simulink model "CrCtl_Governor"  (R2016b)
settings: configuration reference "CodeGenConfigSet" (kept outside this file)
values from neighbouring files (symbols this model uses):
  ACC_ZERO = fi(0,Acc_m_s2)    [init_CrCtl_Governor.m]
  CrCtl_facAcc2TrqCor_C = Calibration.Parameter    [init_CrCtl_Governor.m]
  CrCtl_facDecl2TrqCor_C = Calibration.Parameter    [init_CrCtl_Governor.m]
  CrCtl_facPT11_C = Calibration.Parameter    [init_CrCtl_Governor.m]
  CrCtl_facPT12_C = Calibration.Parameter    [init_CrCtl_Governor.m]
  CrCtl_facPT13_C = Calibration.Parameter    [init_CrCtl_Governor.m]
  CrCtl_facRmpSlpHiAcc_C = Calibration.Parameter    [init_CrCtl_Governor.m]
  CrCtl_facRmpSlpHiDecl_C = Calibration.Parameter    [init_CrCtl_Governor.m]
  CrCtl_facSlpConstRmpDwn_C = Calibration.Parameter    [init_CrCtl_Governor.m]
  CrCtl_facSlpConstRmpUp_C = Calibration.Parameter    [init_CrCtl_Governor.m]
  CrCtl_facSlpRmp1Sus_C = Calibration.Parameter    [init_CrCtl_Governor.m]
  CrCtl_facSlpRmp2Sus_C = Calibration.Parameter    [init_CrCtl_Governor.m]
  CrCtl_facTipDwnCor_CUR = Calibration.Parameter    [init_CrCtl_Governor.m]
  CrCtl_facTipDwnCor_CURX = Calibration.Parameter    [init_CrCtl_Governor.m]
  CrCtl_facTipUpCor_CUR = Calibration.Parameter    [init_CrCtl_Governor.m]
  CrCtl_facTipUpCor_CURX = Calibration.Parameter    [init_CrCtl_Governor.m]
  CrCtl_facTrqIncrSlpConstRmp_C = Calibration.Parameter    [init_CrCtl_Governor.m]
  CrCtl_facTrqIncrTimeConstRmp_C = Calibration.Parameter    [init_CrCtl_Governor.m]
  CrCtl_facTrqRedSlpConstRmp_C = Calibration.Parameter    [init_CrCtl_Governor.m]
  CrCtl_facTrqRedTimeConstRmp_C = Calibration.Parameter    [init_CrCtl_Governor.m]
  CrCtl_facTrqStrtAcc_C = Calibration.Parameter    [init_CrCtl_Governor.m]
  CrCtl_KiAcc1IWin_C = Calibration.Parameter    [init_CrCtl_Governor.m]
  CrCtl_KiAcc2IWin_C = Calibration.Parameter    [init_CrCtl_Governor.m]
  CrCtl_KiAcc3IWin_C = Calibration.Parameter    [init_CrCtl_Governor.m]
  CrCtl_KiCruise1IWin_C = Calibration.Parameter    [init_CrCtl_Governor.m]
  CrCtl_KiCruise2IWin_C = Calibration.Parameter    [init_CrCtl_Governor.m]
  CrCtl_KiCruise3IWin_C = Calibration.Parameter    [init_CrCtl_Governor.m]
  CrCtl_KiDecl1IWin_C = Calibration.Parameter    [init_CrCtl_Governor.m]
  CrCtl_KiDecl2IWin_C = Calibration.Parameter    [init_CrCtl_Governor.m]
  CrCtl_KiDecl3IWin_C = Calibration.Parameter    [init_CrCtl_Governor.m]
  CrCtl_KiNegAcc1IWin_C = Calibration.Parameter    [init_CrCtl_Governor.m]
  CrCtl_KiNegAcc2IWin_C = Calibration.Parameter    [init_CrCtl_Governor.m]
  CrCtl_KiNegAcc3IWin_C = Calibration.Parameter    [init_CrCtl_Governor.m]
  CrCtl_KiNegCruise1IWin_C = Calibration.Parameter    [init_CrCtl_Governor.m]
  CrCtl_KiNegCruise2IWin_C = Calibration.Parameter    [init_CrCtl_Governor.m]
  CrCtl_KiNegCruise3IWin_C = Calibration.Parameter    [init_CrCtl_Governor.m]
  CrCtl_KiNegDecl1IWin_C = Calibration.Parameter    [init_CrCtl_Governor.m]
  CrCtl_KiNegDecl2IWin_C = Calibration.Parameter    [init_CrCtl_Governor.m]
  CrCtl_KiNegDecl3IWin_C = Calibration.Parameter    [init_CrCtl_Governor.m]
  CrCtl_KiNegRes1IWin_C = Calibration.Parameter    [init_CrCtl_Governor.m]
  CrCtl_KiNegRes2IWin_C = Calibration.Parameter    [init_CrCtl_Governor.m]
  CrCtl_KiNegRes3IWin_C = Calibration.Parameter    [init_CrCtl_Governor.m]
  CrCtl_KiNegResCruise1IWin_C = Calibration.Parameter    [init_CrCtl_Governor.m]
  CrCtl_KiNegResCruise2IWin_C = Calibration.Parameter    [init_CrCtl_Governor.m]
  CrCtl_KiNegResCruise3IWin_C = Calibration.Parameter    [init_CrCtl_Governor.m]
  CrCtl_KiPosAcc1IWin_C = Calibration.Parameter    [init_CrCtl_Governor.m]
  CrCtl_KiPosAcc2IWin_C = Calibration.Parameter    [init_CrCtl_Governor.m]
  CrCtl_KiPosAcc3IWin_C = Calibration.Parameter    [init_CrCtl_Governor.m]
  CrCtl_KiPosCruise1IWin_C = Calibration.Parameter    [init_CrCtl_Governor.m]
  CrCtl_KiPosCruise2IWin_C = Calibration.Parameter    [init_CrCtl_Governor.m]
  CrCtl_KiPosCruise3IWin_C = Calibration.Parameter    [init_CrCtl_Governor.m]
  CrCtl_KiPosDecl1IWin_C = Calibration.Parameter    [init_CrCtl_Governor.m]
  CrCtl_KiPosDecl2IWin_C = Calibration.Parameter    [init_CrCtl_Governor.m]
  CrCtl_KiPosDecl3IWin_C = Calibration.Parameter    [init_CrCtl_Governor.m]
  CrCtl_KiPosRes1IWin_C = Calibration.Parameter    [init_CrCtl_Governor.m]
  CrCtl_KiPosRes3IWin_C = Calibration.Parameter    [init_CrCtl_Governor.m]
  CrCtl_KiPosResCruise1IWin_C = Calibration.Parameter    [init_CrCtl_Governor.m]
  CrCtl_KiPosResCruise2IWin_C = Calibration.Parameter    [init_CrCtl_Governor.m]
  CrCtl_KiPosResCruise3IWin_C = Calibration.Parameter    [init_CrCtl_Governor.m]
  CrCtl_KiRes1IWin_C = Calibration.Parameter    [init_CrCtl_Governor.m]
  CrCtl_KiRes2IWin_C = Calibration.Parameter    [init_CrCtl_Governor.m]
  CrCtl_KiRes3IWin_C = Calibration.Parameter    [init_CrCtl_Governor.m]
  CrCtl_KiResCruise1IWin_C = Calibration.Parameter    [init_CrCtl_Governor.m]
  CrCtl_KiResCruise2IWin_C = Calibration.Parameter    [init_CrCtl_Governor.m]
  CrCtl_KiResCruise3IWin_C = Calibration.Parameter    [init_CrCtl_Governor.m]
  CrCtl_KpAcc1PWin_C = Calibration.Parameter    [init_CrCtl_Governor.m]
  CrCtl_KpAcc2PWin_C = Calibration.Parameter    [init_CrCtl_Governor.m]
  CrCtl_KpAcc3PWin_C = Calibration.Parameter    [init_CrCtl_Governor.m]
  CrCtl_KpCruise1PWin_C = Calibration.Parameter    [init_CrCtl_Governor.m]
  CrCtl_KpCruise2PWin_C = Calibration.Parameter    [init_CrCtl_Governor.m]
  CrCtl_KpCruise3PWin_C = Calibration.Parameter    [init_CrCtl_Governor.m]
  CrCtl_KpDecl1PWin_C = Calibration.Parameter    [init_CrCtl_Governor.m]
  CrCtl_KpDecl2PWin_C = Calibration.Parameter    [init_CrCtl_Governor.m]
  CrCtl_KpDecl3PWin_C = Calibration.Parameter    [init_CrCtl_Governor.m]
  CrCtl_KpNegAcc1PWin_C = Calibration.Parameter    [init_CrCtl_Governor.m]
  CrCtl_KpNegAcc2PWin_C = Calibration.Parameter    [init_CrCtl_Governor.m]
  CrCtl_KpNegAcc3PWin_C = Calibration.Parameter    [init_CrCtl_Governor.m]
  CrCtl_KpNegCruise1PWin_C = Calibration.Parameter    [init_CrCtl_Governor.m]
  CrCtl_KpNegCruise2PWin_C = Calibration.Parameter    [init_CrCtl_Governor.m]
  CrCtl_KpNegCruise3PWin_C = Calibration.Parameter    [init_CrCtl_Governor.m]
  CrCtl_KpNegDecl1PWin_C = Calibration.Parameter    [init_CrCtl_Governor.m]
  CrCtl_KpNegDecl2PWin_C = Calibration.Parameter    [init_CrCtl_Governor.m]
  CrCtl_KpNegDecl3PWin_C = Calibration.Parameter    [init_CrCtl_Governor.m]
  CrCtl_KpNegRes1PWin_C = Calibration.Parameter    [init_CrCtl_Governor.m]
  CrCtl_KpNegRes2PWin_C = Calibration.Parameter    [init_CrCtl_Governor.m]
  CrCtl_KpNegRes3PWin_C = Calibration.Parameter    [init_CrCtl_Governor.m]
  CrCtl_KpNegResCruise1PWin_C = Calibration.Parameter    [init_CrCtl_Governor.m]
  CrCtl_KpNegResCruise2PWin_C = Calibration.Parameter    [init_CrCtl_Governor.m]
  CrCtl_KpNegResCruise3PWin_C = Calibration.Parameter    [init_CrCtl_Governor.m]
  CrCtl_KpPosAcc1PWin_C = Calibration.Parameter    [init_CrCtl_Governor.m]
  CrCtl_KpPosAcc2PWin_C = Calibration.Parameter    [init_CrCtl_Governor.m]
  CrCtl_KpPosAcc3PWin_C = Calibration.Parameter    [init_CrCtl_Governor.m]
  CrCtl_KpPosCruise1PWin_C = Calibration.Parameter    [init_CrCtl_Governor.m]
  CrCtl_KpPosCruise2PWin_C = Calibration.Parameter    [init_CrCtl_Governor.m]
  CrCtl_KpPosCruise3PWin_C = Calibration.Parameter    [init_CrCtl_Governor.m]
  CrCtl_KpPosDecl1PWin_C = Calibration.Parameter    [init_CrCtl_Governor.m]
  CrCtl_KpPosDecl2PWin_C = Calibration.Parameter    [init_CrCtl_Governor.m]
  CrCtl_KpPosDecl3PWin_C = Calibration.Parameter    [init_CrCtl_Governor.m]
  CrCtl_KpPosRes1PWin_C = Calibration.Parameter    [init_CrCtl_Governor.m]
  CrCtl_KpPosRes2PWin_C = Calibration.Parameter    [init_CrCtl_Governor.m]
  CrCtl_KpPosRes3PWin_C = Calibration.Parameter    [init_CrCtl_Governor.m]
  CrCtl_KpPosResCruise1PWin_C = Calibration.Parameter    [init_CrCtl_Governor.m]
  CrCtl_KpPosResCruise2PWin_C = Calibration.Parameter    [init_CrCtl_Governor.m]
  CrCtl_KpPosResCruise3PWin_C = Calibration.Parameter    [init_CrCtl_Governor.m]
  CrCtl_KpRes1PWin_C = Calibration.Parameter    [init_CrCtl_Governor.m]
  CrCtl_KpRes2PWin_C = Calibration.Parameter    [init_CrCtl_Governor.m]
  CrCtl_KpRes3PWin_C = Calibration.Parameter    [init_CrCtl_Governor.m]
  CrCtl_KpResCruise1PWin_C = Calibration.Parameter    [init_CrCtl_Governor.m]
  CrCtl_KpResCruise2PWin_C = Calibration.Parameter    [init_CrCtl_Governor.m]
  CrCtl_KpResCruise3PWin_C = Calibration.Parameter    [init_CrCtl_Governor.m]
  CrCtl_numParSelThres1_C = Calibration.Parameter    [init_CrCtl_Governor.m]
  CrCtl_numParSelThres2_C = Calibration.Parameter    [init_CrCtl_Governor.m]
  CrCtl_swtBrkMode_C = Calibration.Parameter    [init_CrCtl_Governor.m]
  CrCtl_swtILimWithP_C = Calibration.Parameter    [init_CrCtl_Governor.m]
  CrCtl_swtOvrRdeFrzInteg_C = Calibration.Parameter    [init_CrCtl_Governor.m]
  CrCtl_swtParSelHysBrk_C = Calibration.Parameter    [init_CrCtl_Governor.m]
  CrCtl_swtPT1EngBrk_C = Calibration.Parameter    [init_CrCtl_Governor.m]
  CrCtl_swtSusRmpInit_C = Calibration.Parameter    [init_CrCtl_Governor.m]
  CrCtl_swtSusRmpStp_C = Calibration.Parameter    [init_CrCtl_Governor.m]
  CrCtl_swtTipUpDwnGvnrStrtVal_C = Calibration.Parameter    [init_CrCtl_Governor.m]
  ... (+88 more)
undefined symbols (not defined in the file or in its folder): CrCtl_Governor_DT, CrCtl_stLck_conv, CrCtl_stOpFunc_conv, CrCtl_stShOff_conv, CrCtl_stSub_conv, CrCtl_stSuspRamp_conv, CruiseCtl_State_conv, EBrk_stPreSelMode_conv, WESDem_State_conv
libraries: CXLib x126, simulink x25
(part 3 of 6)

== system CrCtl_Governor/Deceleration State/CRCTL_SUBSETEND ==
  WESDem_stCurr : Inport
  PT_trqWhl : Inport  Port=2
  CrCtl_trqReq_Old : Inport  Port=3
  Enable : EnablePort
  Constant : Constant  Value=WESDem_State_conv.WESDEM_STOFF
  Relational Operator : RelationalOperator  Operator=~=  OutDataTypeStr=boolean  RndMeth=Simplest
  Switch : Switch  Criteria=u2 ~= 0
  CrCtl_trqReq : Outport
  wires:
  WESDem_stCurr/1 -> Relational Operator/1
  Constant/1 -> Relational Operator/2
  Relational Operator/1 -> Switch/2
  PT_trqWhl/1 -> Switch/1
  Switch/1 -> CrCtl_trqReq/1
  CrCtl_trqReq_Old/1 -> Switch/3

== system CrCtl_Governor/Deceleration State/CRCTL_SUBSTRTVAL ==
  VMD_trqDes : Inport
  PT_rTraV2N : Inport  Port=2
  CrCtl_trqLimAct : Inport  Port=3
  CrCtl_trqMin : Inport  Port=4
  Enable : EnablePort
  Saturation_S16 : CXLib/Saturation_S16
  Terminator : Terminator
  CrCtl_rTraV2NBeg : Outport
  CrCtl_trqReq : Outport  Port=2
  wires:
  PT_rTraV2N/1 -> CrCtl_rTraV2NBeg/1
  CrCtl_trqLimAct/1 -> Saturation_S16/3
  CrCtl_trqMin/1 -> Saturation_S16/2
  VMD_trqDes/1 -> Saturation_S16/1
  Saturation_S16/1 -> CrCtl_trqReq/1
  Saturation_S16/2 -> Terminator/1

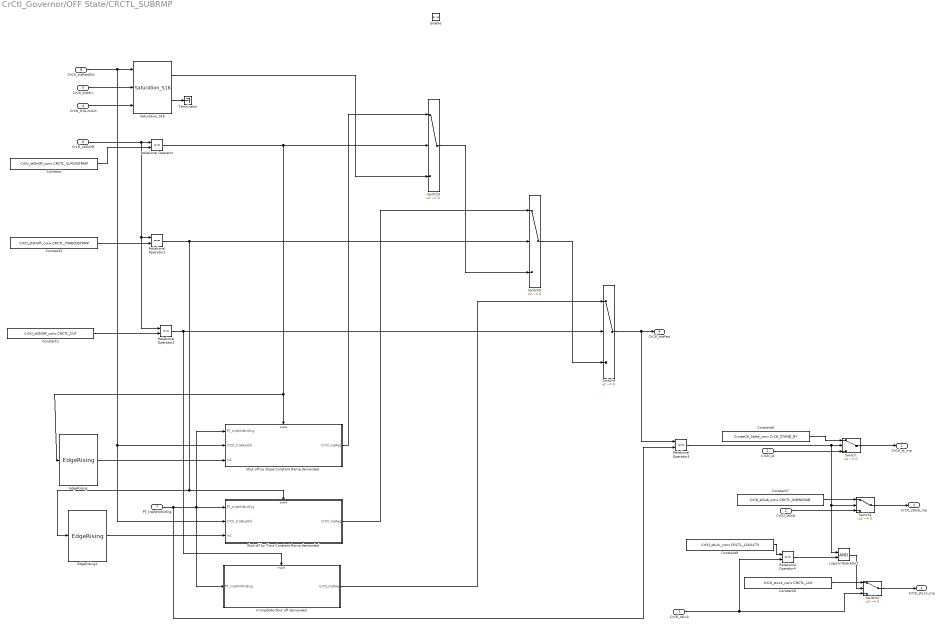
== system CrCtl_Governor/OFF State/CRCTL_SUBRMP ==
  CrCtl_st : Inport
  CrCtl_stSub : Inport  Port=2
  CrCtl_stLck : Inport  Port=3
  CrCtl_trqLimAct : Inport  Port=4
  CrCtl_trqMin : Inport  Port=5
  CrCtl_stShOff : Inport  Port=6
  PT_trqWhlMinEng : Inport  Port=7
  CrCtl_trqReqOld : Inport  Port=8
  Enable : EnablePort
  Constant : Constant  Value=CrCtl_stShOff_conv.CRCTL_SLPCNSTRMP
  Constant1 : Constant  Value=CrCtl_stShOff_conv.CRCTL_TIMECNSTRMP
  Constant2 : Constant  Value=CrCtl_stShOff_conv.CRCTL_CUT
  Constant6 : Constant  Value=CruiseCtl_State_conv.CrCtl_STAND_BY
  Constant7 : Constant  Value=CrCtl_stSub_conv.CRCTL_SUBNOSUB
  Constant8 : Constant  Value=CrCtl_stLck_conv.CRCTL_LCK
  Constant9 : Constant  Value=CrCtl_stLck_conv.CRCTL_LCKACTV
  EdgeRising : CXLib/EdgeRising
  EdgeRising1 : CXLib/EdgeRising
  Immediate Shut off demanded : Subsystem
  Logical Operator2 : Logic  AllPortsSameDT=off  OutDataTypeStr=boolean
  Relational Operator{,1..4} (5 alike) : RelationalOperator  Operator===  OutDataTypeStr=boolean  RndMeth=Simplest
  Saturation_S16 : CXLib/Saturation_S16
  Shut off by Slope Constant Ramp demanded : Subsystem
  Shut off by Time Constant Ramp demanded : Subsystem
  Switch{,1..5} (6 alike) : Switch  Criteria=u2 ~= 0
  Terminator : Terminator
  CrCtl_st_mp : Outport
  CrCtl_stSub_mp : Outport  Port=2
  CrCtl_stLck_mp : Outport  Port=3
  CrCtl_trqReq : Outport  Port=4
  wires:
  Constant6/1 -> Switch/1
  Switch/1 -> CrCtl_st_mp/1
  Relational Operator3/1 -> Switch1/2, Logical Operator2/1, Switch/2
  Constant7/1 -> Switch1/1
  Switch1/1 -> CrCtl_stSub_mp/1
  Logical Operator2/1 -> Switch2/2
  CrCtl_stLck/1 -> Switch2/3, Relational Operator4/2
  Constant8/1 -> Switch2/1
  Switch2/1 -> CrCtl_stLck_mp/1
  Relational Operator4/1 -> Logical Operator2/2
  Constant9/1 -> Relational Operator4/1
  CrCtl_st/1 -> Switch/3
  CrCtl_stSub/1 -> Switch1/3
  CrCtl_trqMin/1 -> Saturation_S16/2
  CrCtl_trqLimAct/1 -> Saturation_S16/3
  Saturation_S16/2 -> Terminator/1
  CrCtl_trqReqOld/1 -> Shut off by Time Constant Ramp demanded/2(CrCtl_trqReqOld), Shut off by Slope Constant Ramp demanded/2(CrCtl_trqReqOld), Saturation_S16/1
  CrCtl_stShOff/1 -> Relational Operator2/1, Relational Operator1/1, Relational Operator/1
  Constant/1 -> Relational Operator/2
  Constant1/1 -> Relational Operator1/2
  Constant2/1 -> Relational Operator2/2
  Relational Operator/1 -> EdgeRising/1, Shut off by Slope Constant Ramp demanded/Enable, Switch3/2
  Relational Operator1/1 -> EdgeRising1/1, Shut off by Time Constant Ramp demanded/Enable, Switch5/2
  Relational Operator2/1 -> Immediate Shut off demanded/Enable, Switch4/2
  Switch4/1 -> Relational Operator3/1, CrCtl_trqReq/1
  Switch5/1 -> Switch4/3
  Immediate Shut off demanded/1(CrCtl_trqReq) -> Switch4/1
  Shut off by Time Constant Ramp demanded/1(CrCtl_trqReq) -> Switch5/1
  Switch3/1 -> Switch5/3
  Saturation_S16/1 -> Switch3/3
  Shut off by Slope Constant Ramp demanded/1(CrCtl_trqReq) -> Switch3/1
  EdgeRising/1 -> Shut off by Slope Constant Ramp demanded/3(In1)
  EdgeRising1/1 -> Shut off by Time Constant Ramp demanded/3(In1)
  PT_trqWhlMinEng/1 -> Relational Operator3/2, Immediate Shut off demanded/1(PT_trqWhlMinEng), Shut off by Time Constant Ramp demanded/1(PT_trqWhlMinEng), Shut off by Slope Constant Ramp demanded/1(PT_trqWhlMinEng)

== system CrCtl_Governor/OFF State/CRCTL_SUBSTRTVAL  ==
  CrCtl_trqLimAct : Inport
  CrCtl_trqMin : Inport  Port=2
  CrCtl_trqReqOld : Inport  Port=3
  Enable : EnablePort
  Saturation_S16 : CXLib/Saturation_S16
  Terminator : Terminator
  CrCtl_trqReq : Outport
  wires:
  CrCtl_trqMin/1 -> Saturation_S16/2
  CrCtl_trqLimAct/1 -> Saturation_S16/3
  Saturation_S16/2 -> Terminator/1
  CrCtl_trqReqOld/1 -> Saturation_S16/1
  Saturation_S16/1 -> CrCtl_trqReq/1

== system CrCtl_Governor/Resume From Above/CRCTL_SUBRMP ==
  GlbDa_vXFlt : Inport
  CrCtl_trqLimAct : Inport  Port=2
  CrCtl_trqMin : Inport  Port=3
  CrCtl_vDesAct : Inport  Port=4
  stvHysEngBrkReq : Inport  Port=5
  APP_r : Inport  Port=6
  AccPed_trqDes : Inport  Port=7
  CrCtl_vDes : Inport  Port=8
  CrCtl_trqReqOld : Inport  Port=9
  PT_trqWhlMinEng : Inport  Port=10
  CrCtl_stGearRng_mp : Inport  Port=11
  stCrCtlOn : Inport  Port=12
  CrCtl_stSuspAct : Inport  Port=13
  In2 : Inport  Port=14
  Enable : EnablePort
  Constant1 : Constant  Value=0  OutDataTypeStr=uint8
  Constant3 : Constant  Value=0  OutDataTypeStr=uint8
  CrCtl_OverRide : Subsystem
  CrCtl_Suspend : Subsystem
  Data Type Conversion : DataTypeConversion  OutDataTypeStr=uint8
  Data Type Conversion1 : DataTypeConversion  OutDataTypeStr=uint8
  EdgeRising : CXLib/EdgeRising
  Governor : Subsystem
  Relational Operator1 : RelationalOperator  Operator===  OutDataTypeStr=boolean  RndMeth=Simplest
  Relational Operator2 : RelationalOperator  Operator=~=  OutDataTypeStr=boolean  RndMeth=Simplest
  Switch : Switch  Criteria=u2 ~= 0
  Unit Delay : UnitDelay  InitialCondition=CrCtl_stSuspRamp_conv.CRCTL_SUSPENDNOTACTIVE  SampleTime=-1
  Unit Delay2 : UnitDelay  SampleTime=-1
  CrCtl_stSuspRamp : Outport
  CrCtl_trqReq : Outport  Port=2
  CrCtl_stIWin_mp : Outport  Port=3
  CrCtl_trqReqIWin_mp : Outport  Port=4
  CrCtl_trqReqPWin_mp : Outport  Port=5
  wires:
  Constant3/1 -> Relational Operator1/2
  stCrCtlOn/1 -> Governor/7(stCrCtlOn)
  stvHysEngBrkReq/1 -> Governor/5(stvHysEngBrkReq)
  CrCtl_vDesAct/1 -> Governor/4(CrCtl_vDesAct)
  CrCtl_stGearRng_mp/1 -> Governor/3(CrCtl_stGearRng_mp)
  CrCtl_trqMin/1 -> Governor/2(CrCtl_trqMin), CrCtl_OverRide/2(CrCtl_trqMin)
  APP_r/1 -> CrCtl_OverRide/3(APP_r)
  CrCtl_vDes/1 -> CrCtl_OverRide/5(CrCtl_vDes)
  GlbDa_vXFlt/1 -> Governor/6(GlbDa_vXFlt), CrCtl_OverRide/6(GlbDa_vXFlt)
  Governor/1(CrCtl_trqReq) -> Switch/3, CrCtl_OverRide/7(CrCtl_trqReq)
  Governor/2(CrCtl_trqIWinOld_mp) -> CrCtl_OverRide/8(CrCtl_trqIWinOld_mp)
  CrCtl_trqLimAct/1 -> Governor/1(CrCtl_trqLimAct), CrCtl_Suspend/4(CrCtl_trqLimAct), CrCtl_OverRide/1(CrCtl_trqLimAct)
  AccPed_trqDes/1 -> CrCtl_Suspend/3(AccPed_trqDes), CrCtl_OverRide/4(AccPed_trqDes)
  PT_trqWhlMinEng/1 -> CrCtl_Suspend/1(PT_trqWhlMinEng)
  CrCtl_trqReqOld/1 -> CrCtl_Suspend/2(CrCtl_trqReqOld)
  CrCtl_stSuspAct/1 -> CrCtl_Suspend/5(CrCtl_stSuspAct)
  CrCtl_Suspend/2(" CrCtl_trqReq") -> Switch/1
  CrCtl_Suspend/1(CrCtl_stSuspRamp) -> Unit Delay/1, Data Type Conversion1/1, CrCtl_stSuspRamp/1
  Switch/1 -> CrCtl_trqReq/1
  Constant1/1 -> Relational Operator2/2
  Relational Operator2/1 -> Unit Delay2/1
  CrCtl_OverRide/1(CrCtl_stIWin_mp) -> CrCtl_stIWin_mp/1
  CrCtl_OverRide/2(CrCtl_trqReqIWin_mp) -> CrCtl_trqReqIWin_mp/1
  Data Type Conversion/1 -> Relational Operator1/1
  Data Type Conversion1/1 -> Relational Operator2/1
  Unit Delay2/1 -> Switch/2
  Unit Delay/1 -> Data Type Conversion/1
  Governor/3(CrCtl_trqReqPWin_mp) -> CrCtl_trqReqPWin_mp/1
  Relational Operator1/1 -> EdgeRising/1, Governor/Enable
  EdgeRising/1 -> Governor/8(In1)
  In2/1 -> Governor/9(In2)

== system CrCtl_Governor/Resume From Above/CRCTL_SUBSTRTVAL ==
  PT_rTraV2N : Inport
  WESDem_stCurr : Inport  Port=2
  VMD_trqDes : Inport  Port=3
  GlbDa_vXFlt : Inport  Port=4
  CrCtl_GearRng_mp : Inport  Port=5
  CrCtl_vDesAct : Inport  Port=6
  PT_trqWhl : Inport  Port=7
  CrCtl_trqMin : Inport  Port=8
  CrCtl_trqLimAct : Inport  Port=9
  Enable : EnablePort
  Add : Sum  Inputs=+-
  Add1 : Sum  Inputs=+-
  Add2 : Sum  Inputs=+-
  Add3 : Sum  Inputs=+-  OutDataTypeStr=Trq_Nm
  Constant : Constant  Value=WESDem_State_conv.WESDEM_STOFF
  Constant1 : Constant  Value=CrCtl_trqOfsResAbv_C
  CrCtl_trqVCorResAbv_CUR : Lookup_n-D  NumberOfTableDimensions=1  BreakpointsForDimension1=CrCtl_trqVCorResAbv_CURX  Table=CrCtl_trqVCorResAbv_CUR  ExtrapMethod=Clip  InternalRulePriority=Speed  OutDataTypeStr=Inherit: Inherit via back propagation  RndMeth=Simplest  InputSameDT=on
  P_S16 : CXLib/P_S16
  Parameter Selection for Kp : Subsystem
  Relational Operator : RelationalOperator  Operator=~=  OutDataTypeStr=boolean  RndMeth=Simplest
  Saturation_S16 : CXLib/Saturation_S16
  Switch2 : Switch  Criteria=u2 ~= 0
  Terminator : Terminator
  CrCtl_rTraV2NBeg : Outport
  CrCtl_trqReqIWin_mp : Outport  Port=2
  CrCtl_trqReq : Outport  Port=3
  wires:
  PT_rTraV2N/1 -> CrCtl_rTraV2NBeg/1
  Constant/1 -> Relational Operator/2
  WESDem_stCurr/1 -> Relational Operator/1
  VMD_trqDes/1 -> Add/1
  Relational Operator/1 -> Switch2/2
  PT_trqWhl/1 -> Switch2/1
  GlbDa_vXFlt/1 -> CrCtl_trqVCorResAbv_CUR/1, Add2/2
  CrCtl_trqVCorResAbv_CUR/1 -> Add/2
  CrCtl_vDesAct/1 -> Add2/1
  CrCtl_GearRng_mp/1 -> Parameter Selection for Kp/1(CrCtl_stGearRng_mp)
  Parameter Selection for Kp/2(Out2) -> P_S16/3
  Parameter Selection for Kp/3(Out3) -> P_S16/4
  Parameter Selection for Kp/4(Out4) -> P_S16/5
  Add2/1 -> P_S16/1
  Parameter Selection for Kp/1(Out1) -> P_S16/2
  Parameter Selection for Kp/5(Out5) -> P_S16/6
  CrCtl_trqMin/1 -> Saturation_S16/2
  CrCtl_trqLimAct/1 -> Saturation_S16/3
  Switch2/1 -> Saturation_S16/1
  Saturation_S16/1 -> CrCtl_trqReq/1, Add3/1
  P_S16/1 -> Add3/2
  Add3/1 -> CrCtl_trqReqIWin_mp/1
  Add/1 -> Add1/1
  Constant1/1 -> Add1/2
  Add1/1 -> Switch2/3
  Saturation_S16/2 -> Terminator/1

== system CrCtl_Governor/Resume From Below/CRCTL_SUBPRECRUISE ==
  GlbDa_vXFlt : Inport
  CrCtl_trqLimAct : Inport  Port=2
  CrCtl_trqMin : Inport  Port=3
  CrCtl_vDesAct : Inport  Port=4
  stvHysEngBrkReq : Inport  Port=5
  APP_r : Inport  Port=6
  AccPed_trqDes : Inport  Port=7
  CrCtl_vDes : Inport  Port=8
  CrCtl_trqReqOld : Inport  Port=9
  PT_trqWhlMinEng : Inport  Port=10
  CrCtl_stGearRng_mp : Inport  Port=11
  stCrCtlOn : Inport  Port=12
  CrCtl_stSuspAct : Inport  Port=13
  In2 : Inport  Port=14
  Enable : EnablePort
  Constant1 : Constant  Value=0  OutDataTypeStr=uint8
  Constant2 : Constant  Value=0  OutDataTypeStr=uint8
  CrCtl_OverRide : Subsystem
  CrCtl_Suspend : Subsystem
  Data Type Conversion : DataTypeConversion  OutDataTypeStr=uint8
  Data Type Conversion1 : DataTypeConversion  OutDataTypeStr=uint8
  EdgeRising : CXLib/EdgeRising
  Governor : Subsystem
  Relational Operator1 : RelationalOperator  Operator===  OutDataTypeStr=boolean  RndMeth=Simplest
  Relational Operator2 : RelationalOperator  Operator=~=  OutDataTypeStr=boolean  RndMeth=Simplest
  Switch : Switch  Criteria=u2 ~= 0
  Unit Delay : UnitDelay  InitialCondition=CrCtl_stSuspRamp_conv.CRCTL_SUSPENDNOTACTIVE  SampleTime=-1
  Unit Delay2 : UnitDelay  SampleTime=-1
  CrCtl_stSuspRamp : Outport
  CrCtl_trqReq : Outport  Port=2
  CrCtl_stIWin_mp : Outport  Port=3
  CrCtl_trqReqIWin_mp : Outport  Port=4
  CrCtl_trqReqPWin_mp : Outport  Port=5
  wires:
  Constant1/1 -> Relational Operator1/2
  Relational Operator1/1 -> Governor/Enable, EdgeRising/1
  stCrCtlOn/1 -> Governor/7(stCrCtlOn)
  stvHysEngBrkReq/1 -> Governor/5(stvHysEngBrkReq)
  CrCtl_vDesAct/1 -> Governor/4(CrCtl_vDesAct)
  CrCtl_stGearRng_mp/1 -> Governor/3(CrCtl_stGearRng_mp)
  CrCtl_trqMin/1 -> Governor/2(CrCtl_trqMin), CrCtl_OverRide/2(CrCtl_trqMin)
  APP_r/1 -> CrCtl_OverRide/3(APP_r)
  CrCtl_vDes/1 -> CrCtl_OverRide/5(CrCtl_vDes)
  GlbDa_vXFlt/1 -> Governor/6(GlbDa_vXFlt), CrCtl_OverRide/6(GlbDa_vXFlt)
  Governor/1(CrCtl_trqReq) -> Switch/3, CrCtl_OverRide/7(CrCtl_trqReq)
  Governor/2(CrCtl_trqIWinOld_mp) -> CrCtl_OverRide/8(CrCtl_trqIWinOld_mp)
  CrCtl_trqLimAct/1 -> Governor/1(CrCtl_trqLimAct), CrCtl_Suspend/4(CrCtl_trqLimAct), CrCtl_OverRide/1(CrCtl_trqLimAct)
  AccPed_trqDes/1 -> CrCtl_Suspend/3(AccPed_trqDes), CrCtl_OverRide/4(AccPed_trqDes)
  PT_trqWhlMinEng/1 -> CrCtl_Suspend/1(PT_trqWhlMinEng)
  CrCtl_trqReqOld/1 -> CrCtl_Suspend/2(CrCtl_trqReqOld)
  CrCtl_stSuspAct/1 -> CrCtl_Suspend/5(CrCtl_stSuspAct)
  CrCtl_Suspend/2(" CrCtl_trqReq") -> Switch/1
  CrCtl_Suspend/1(CrCtl_stSuspRamp) -> Unit Delay/1, Data Type Conversion1/1, CrCtl_stSuspRamp/1
  Switch/1 -> CrCtl_trqReq/1
  Constant2/1 -> Relational Operator2/2
  Relational Operator2/1 -> Unit Delay2/1
  CrCtl_OverRide/1(CrCtl_stIWin_mp) -> CrCtl_stIWin_mp/1
  CrCtl_OverRide/2(CrCtl_trqReqIWin_mp) -> CrCtl_trqReqIWin_mp/1
  Data Type Conversion/1 -> Relational Operator1/1
  Data Type Conversion1/1 -> Relational Operator2/1
  Unit Delay/1 -> Data Type Conversion/1
  Unit Delay2/1 -> Switch/2
  Governor/3(CrCtl_trqReqPWin_mp) -> CrCtl_trqReqPWin_mp/1
  EdgeRising/1 -> Governor/8(In1)
  In2/1 -> Governor/9(In2)

== system CrCtl_Governor/Resume From Below/CRCTL_SUBRMP ==
  GlbDa_vXFlt : Inport
  CrCtl_trqLimAct : Inport  Port=2
  CrCtl_trqMin : Inport  Port=3
  CrCtl_vDesAct : Inport  Port=4
  stvHysEngBrkReq : Inport  Port=5
  APP_r : Inport  Port=6
  AccPed_trqDes : Inport  Port=7
  CrCtl_vDes : Inport  Port=8
  CrCtl_trqReqOld : Inport  Port=9
  PT_trqWhlMinEng : Inport  Port=10
  CrCtl_stGearRng_mp : Inport  Port=11
  stCrCtlOn : Inport  Port=12
  CrCtl_stSuspAct : Inport  Port=13
  In2 : Inport  Port=14
  Enable : EnablePort
  Constant1 : Constant  Value=0  OutDataTypeStr=uint8
  Constant3 : Constant  Value=0  OutDataTypeStr=uint8
  CrCtl_OverRide : Subsystem
  CrCtl_Suspend : Subsystem
  Data Type Conversion : DataTypeConversion  OutDataTypeStr=uint8
  Data Type Conversion1 : DataTypeConversion  OutDataTypeStr=uint8
  EdgeRising : CXLib/EdgeRising
  Governor : Subsystem
  Relational Operator1 : RelationalOperator  Operator===  OutDataTypeStr=boolean  RndMeth=Simplest
  Relational Operator2 : RelationalOperator  Operator=~=  OutDataTypeStr=boolean  RndMeth=Simplest
  Switch : Switch  Criteria=u2 ~= 0
  Unit Delay : UnitDelay  InitialCondition=CrCtl_stSuspRamp_conv.CRCTL_SUSPENDNOTACTIVE  SampleTime=-1
  Unit Delay2 : UnitDelay  SampleTime=-1
  CrCtl_stSuspRamp : Outport
  CrCtl_trqReq : Outport  Port=2
  CrCtl_stIWin_mp : Outport  Port=3
  CrCtl_trqReqIWin_mp : Outport  Port=4
  CrCtl_trqReqPWin_mp : Outport  Port=5
  wires:
  Constant3/1 -> Relational Operator1/2
  stCrCtlOn/1 -> Governor/7(stCrCtlOn)
  stvHysEngBrkReq/1 -> Governor/5(stvHysEngBrkReq)
  CrCtl_vDesAct/1 -> Governor/4(CrCtl_vDesAct)
  CrCtl_stGearRng_mp/1 -> Governor/3(CrCtl_stGearRng_mp)
  CrCtl_trqMin/1 -> Governor/2(CrCtl_trqMin), CrCtl_OverRide/2(CrCtl_trqMin)
  APP_r/1 -> CrCtl_OverRide/3(APP_r)
  CrCtl_vDes/1 -> CrCtl_OverRide/5(CrCtl_vDes)
  GlbDa_vXFlt/1 -> Governor/6(GlbDa_vXFlt), CrCtl_OverRide/6(GlbDa_vXFlt)
  Governor/1(CrCtl_trqReq) -> Switch/3, CrCtl_OverRide/7(CrCtl_trqReq)
  Governor/2(CrCtl_trqIWinOld_mp) -> CrCtl_OverRide/8(CrCtl_trqIWinOld_mp)
  CrCtl_trqLimAct/1 -> Governor/1(CrCtl_trqLimAct), CrCtl_Suspend/4(CrCtl_trqLimAct), CrCtl_OverRide/1(CrCtl_trqLimAct)
  AccPed_trqDes/1 -> CrCtl_Suspend/3(AccPed_trqDes), CrCtl_OverRide/4(AccPed_trqDes)
  PT_trqWhlMinEng/1 -> CrCtl_Suspend/1(PT_trqWhlMinEng)
  CrCtl_trqReqOld/1 -> CrCtl_Suspend/2(CrCtl_trqReqOld)
  CrCtl_stSuspAct/1 -> CrCtl_Suspend/5(CrCtl_stSuspAct)
  CrCtl_Suspend/2(" CrCtl_trqReq") -> Switch/1
  CrCtl_Suspend/1(CrCtl_stSuspRamp) -> Unit Delay/1, Data Type Conversion1/1, CrCtl_stSuspRamp/1
  Switch/1 -> CrCtl_trqReq/1
  Constant1/1 -> Relational Operator2/2
  Relational Operator2/1 -> Unit Delay2/1
  CrCtl_OverRide/1(CrCtl_stIWin_mp) -> CrCtl_stIWin_mp/1
  CrCtl_OverRide/2(CrCtl_trqReqIWin_mp) -> CrCtl_trqReqIWin_mp/1
  Data Type Conversion/1 -> Relational Operator1/1
  Data Type Conversion1/1 -> Relational Operator2/1
  Unit Delay2/1 -> Switch/2
  Unit Delay/1 -> Data Type Conversion/1
  Governor/3(CrCtl_trqReqPWin_mp) -> CrCtl_trqReqPWin_mp/1
  Relational Operator1/1 -> EdgeRising/1, Governor/Enable
  EdgeRising/1 -> Governor/8(In1)
  In2/1 -> Governor/9(In2)

== system CrCtl_Governor/Resume From Below/CRCTL_SUBSTRTVAL ==
  PT_rTraV2N : Inport
  WESDem_stCurr : Inport  Port=2
  VMD_trqDes : Inport  Port=3
  GlbDa_vXFlt : Inport  Port=4
  CrCtl_stGearRng_mp : Inport  Port=5
  CrCtl_vDesAct : Inport  Port=6
  PT_trqWhl : Inport  Port=7
  CrCtl_trqMin : Inport  Port=8
  CrCtl_trqLimAct : Inport  Port=9
  Enable : EnablePort
  Add : Sum
  Add1 : Sum
  Add2 : Sum  Inputs=+-
  Add3 : Sum  Inputs=+-  OutDataTypeStr=Trq_Nm
  Constant : Constant  Value=WESDem_State_conv.WESDEM_STOFF
  Constant1 : Constant  Value=CrCtl_trqOfsResBlw_C
  CrCtl_trqVCorResBlw_CUR : Lookup_n-D  NumberOfTableDimensions=1  BreakpointsForDimension1=CrCtl_trqVCorResBlw_CURX  Table=CrCtl_trqVCorResBlw_CUR  ExtrapMethod=Clip  InternalRulePriority=Speed  OutDataTypeStr=Inherit: Inherit via back propagation  RndMeth=Simplest  InputSameDT=on
  P_S16 : CXLib/P_S16
  Parameter Selection for Kp : Subsystem
  Relational Operator : RelationalOperator  Operator=~=  OutDataTypeStr=boolean  RndMeth=Simplest
  Saturation_S16 : CXLib/Saturation_S16
  Switch2 : Switch  Criteria=u2 ~= 0
  Terminator : Terminator
  CrCtl_rTraV2NBeg : Outport
  CrCtl_trqReqIWin_mp : Outport  Port=2
  CrCtl_trqReq : Outport  Port=3
  wires:
  PT_rTraV2N/1 -> CrCtl_rTraV2NBeg/1
  Constant/1 -> Relational Operator/2
  WESDem_stCurr/1 -> Relational Operator/1
  VMD_trqDes/1 -> Add/1
  Relational Operator/1 -> Switch2/2
  PT_trqWhl/1 -> Switch2/1
  GlbDa_vXFlt/1 -> CrCtl_trqVCorResBlw_CUR/1, Add2/2
  CrCtl_trqVCorResBlw_CUR/1 -> Add/2
  CrCtl_vDesAct/1 -> Add2/1
  CrCtl_stGearRng_mp/1 -> Parameter Selection for Kp/1(CrCtl_stGearRng_mp)
  Parameter Selection for Kp/2(Out2) -> P_S16/3
  Parameter Selection for Kp/3(Out3) -> P_S16/4
  Parameter Selection for Kp/4(Out4) -> P_S16/5
  Add2/1 -> P_S16/1
  Parameter Selection for Kp/1(Out1) -> P_S16/2
  Parameter Selection for Kp/5(Out5) -> P_S16/6
  CrCtl_trqMin/1 -> Saturation_S16/2
  CrCtl_trqLimAct/1 -> Saturation_S16/3
  Saturation_S16/1 -> CrCtl_trqReq/1, Add3/1
  P_S16/1 -> Add3/2
  Add3/1 -> CrCtl_trqReqIWin_mp/1
  Add/1 -> Add1/1
  Constant1/1 -> Add1/2
  Add1/1 -> Switch2/3
  Saturation_S16/2 -> Terminator/1
  Switch2/1 -> Saturation_S16/1

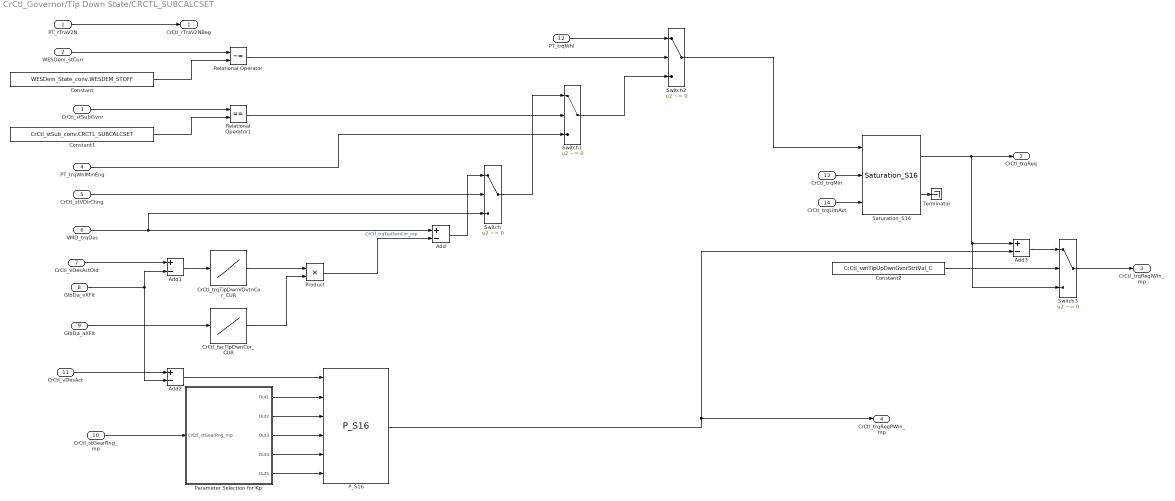
== system CrCtl_Governor/Tip Down State/CRCTL_SUBCALCSET  ==
  PT_rTraV2N : Inport
  WESDem_stCurr : Inport  Port=2
  CrCtl_stSubGvnr : Inport  Port=3
  PT_trqWhlMinEng : Inport  Port=4
  CrCtl_stVDirChng : Inport  Port=5
  VMD_trqDes : Inport  Port=6
  CrCtl_vDesActOld : Inport  Port=7
  GlbDa_vXFlt : Inport  Port=8
  GlbDa_aXFlt : Inport  Port=9
  CrCtl_stGearRng_mp : Inport  Port=10
  CrCtl_vDesAct : Inport  Port=11
  PT_trqWhl : Inport  Port=12
  CrCtl_trqMin : Inport  Port=13
  CrCtl_trqLimAct : Inport  Port=14
  Add : Sum  Inputs=+-
  Add1 : Sum  Inputs=+-
  Add2 : Sum  Inputs=+-
  Add3 : Sum  Inputs=+-  OutDataTypeStr=Trq_Nm
  Constant : Constant  Value=WESDem_State_conv.WESDEM_STOFF
  Constant1 : Constant  Value=CrCtl_stSub_conv.CRCTL_SUBCALCSET
  Constant2 : Constant  Value=CrCtl_swtTipUpDwnGvnrStrtVal_C
  CrCtl_facTipDwnCor_CUR : Lookup_n-D  NumberOfTableDimensions=1  BreakpointsForDimension1=CrCtl_facTipDwnCor_CURX  Table=CrCtl_facTipDwnCor_CUR  ExtrapMethod=Clip  InternalRulePriority=Speed  OutDataTypeStr=Inherit: Inherit via back propagation  RndMeth=Simplest  InputSameDT=on
  CrCtl_trqTipDwnVDvtnCor_CUR : Lookup_n-D  NumberOfTableDimensions=1  BreakpointsForDimension1=CrCtl_trqTipDwnVDvtnCor_CURX  Table=CrCtl_trqTipDwnVDvtnCor_CUR  ExtrapMethod=Clip  InternalRulePriority=Speed  OutDataTypeStr=Inherit: Inherit via back propagation  RndMeth=Simplest  InputSameDT=on
  P_S16 : CXLib/P_S16
  Parameter Selection for Kp : Subsystem
  Product : Product  OutDataTypeStr=Trq_Nm
  Relational Operator : RelationalOperator  Operator=~=  OutDataTypeStr=boolean  RndMeth=Simplest
  Relational Operator1 : RelationalOperator  Operator===  OutDataTypeStr=boolean  RndMeth=Simplest
  Saturation_S16 : CXLib/Saturation_S16
  Switch{,1..3} (4 alike) : Switch  Criteria=u2 ~= 0
  Terminator : Terminator
  CrCtl_rTraV2NBeg : Outport
  CrCtl_trqReq : Outport  Port=2
  CrCtl_trqReqIWin_mp : Outport  Port=3
  CrCtl_trqReqPWin_mp : Outport  Port=4
  wires:
  Saturation_S16/2 -> Terminator/1
  PT_rTraV2N/1 -> CrCtl_rTraV2NBeg/1
  Constant/1 -> Relational Operator/2
  WESDem_stCurr/1 -> Relational Operator/1
  CrCtl_stSubGvnr/1 -> Relational Operator1/1
  Constant1/1 -> Relational Operator1/2
  Relational Operator/1 -> Switch2/2
  VMD_trqDes/1 -> Switch/3, Add/1
  CrCtl_trqMin/1 -> Saturation_S16/2
  Switch2/1 -> Saturation_S16/1
  Constant2/1 -> Switch3/2
  Switch3/1 -> CrCtl_trqReqIWin_mp/1
  Parameter Selection for Kp/4(Out4) -> P_S16/5
  GlbDa_aXFlt/1 -> CrCtl_facTipDwnCor_CUR/1
  CrCtl_vDesActOld/1 -> Add1/1
  Relational Operator1/1 -> Switch1/2
  Switch1/1 -> Switch2/3
  Product/1 -> Add/2  "CrCtl_trqTipDwnCor_mp"
  Add/1 -> Switch/1
  Parameter Selection for Kp/3(Out3) -> P_S16/4
  PT_trqWhl/1 -> Switch2/1
  CrCtl_trqTipDwnVDvtnCor_CUR/1 -> Product/1
  Parameter Selection for Kp/1(Out1) -> P_S16/2
  Parameter Selection for Kp/2(Out2) -> P_S16/3
  CrCtl_stVDirChng/1 -> Switch/2
  Saturation_S16/1 -> CrCtl_trqReq/1, Switch3/3, Add3/1
  GlbDa_vXFlt/1 -> Add1/2, Add2/2
  CrCtl_stGearRng_mp/1 -> Parameter Selection for Kp/1(CrCtl_stGearRng_mp)
  Switch/1 -> Switch1/1
  CrCtl_vDesAct/1 -> Add2/1
  Parameter Selection for Kp/5(Out5) -> P_S16/6
  Add3/1 -> Switch3/1
  CrCtl_trqLimAct/1 -> Saturation_S16/3
  Add1/1 -> CrCtl_trqTipDwnVDvtnCor_CUR/1
  PT_trqWhlMinEng/1 -> Switch1/3
  CrCtl_facTipDwnCor_CUR/1 -> Product/2
  Add2/1 -> P_S16/1
  P_S16/1 -> CrCtl_trqReqPWin_mp/1, Add3/2

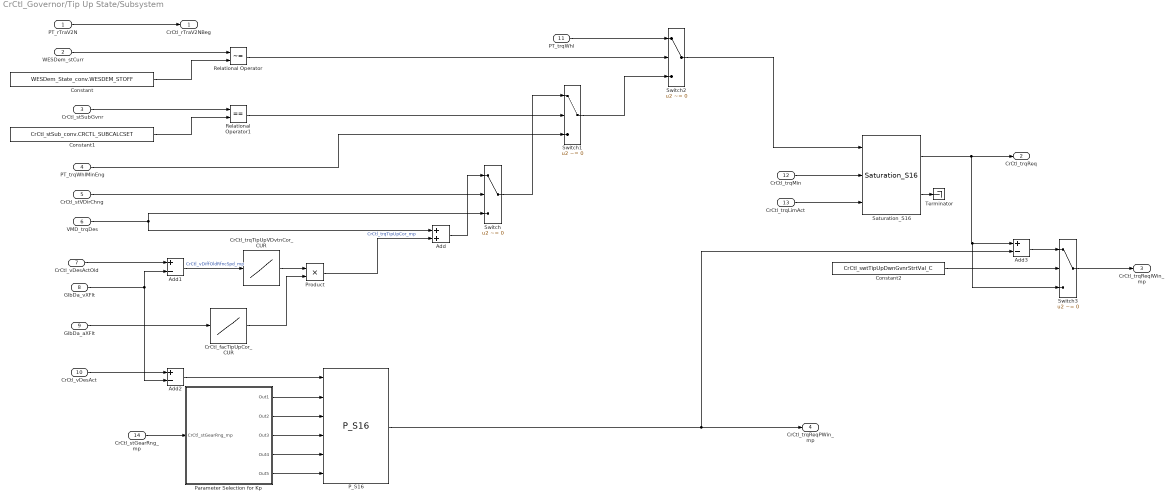
== system CrCtl_Governor/Tip Up State/Subsystem ==
  PT_rTraV2N : Inport
  WESDem_stCurr : Inport  Port=2
  CrCtl_stSubGvnr : Inport  Port=3
  PT_trqWhlMinEng : Inport  Port=4
  CrCtl_stVDirChng : Inport  Port=5
  VMD_trqDes : Inport  Port=6
  CrCtl_vDesActOld : Inport  Port=7
  GlbDa_vXFlt : Inport  Port=8
  GlbDa_aXFlt : Inport  Port=9
  CrCtl_vDesAct : Inport  Port=10
  PT_trqWhl : Inport  Port=11
  CrCtl_trqMin : Inport  Port=12
  CrCtl_trqLimAct : Inport  Port=13
  CrCtl_stGearRng_mp : Inport  Port=14
  Add : Sum
  Add1 : Sum  Inputs=+-
  Add2 : Sum  Inputs=+-
  Add3 : Sum  Inputs=+-  OutDataTypeStr=Trq_Nm
  Constant : Constant  Value=WESDem_State_conv.WESDEM_STOFF
  Constant1 : Constant  Value=CrCtl_stSub_conv.CRCTL_SUBCALCSET
  Constant2 : Constant  Value=CrCtl_swtTipUpDwnGvnrStrtVal_C
  CrCtl_facTipUpCor_CUR : Lookup_n-D  NumberOfTableDimensions=1  BreakpointsForDimension1=CrCtl_facTipUpCor_CURX  Table=CrCtl_facTipUpCor_CUR  ExtrapMethod=Clip  InternalRulePriority=Speed  OutDataTypeStr=Inherit: Inherit via back propagation  RndMeth=Simplest  InputSameDT=on
  CrCtl_trqTipUpVDvtnCor_CUR : Lookup_n-D  NumberOfTableDimensions=1  BreakpointsForDimension1=CrCtl_trqTipUpVDvtnCor_CURX  Table=CrCtl_trqTipUpVDvtnCor_CUR  ExtrapMethod=Clip  InternalRulePriority=Speed  OutDataTypeStr=Inherit: Inherit via back propagation  RndMeth=Simplest  InputSameDT=on
  P_S16 : CXLib/P_S16
  Parameter Selection for Kp : Subsystem
  Product : Product  OutDataTypeStr=Trq_Nm
  Relational Operator : RelationalOperator  Operator=~=  OutDataTypeStr=boolean  RndMeth=Simplest
  Relational Operator1 : RelationalOperator  Operator===  OutDataTypeStr=boolean  RndMeth=Simplest
  Saturation_S16 : CXLib/Saturation_S16
  Switch{,1..3} (4 alike) : Switch  Criteria=u2 ~= 0
  Terminator : Terminator
  CrCtl_rTraV2NBeg : Outport
  CrCtl_trqReq : Outport  Port=2
  CrCtl_trqReqIWin_mp : Outport  Port=3
  CrCtl_trqReqPWin_mp : Outport  Port=4
  wires:
  Saturation_S16/2 -> Terminator/1
  Constant/1 -> Relational Operator/2
  WESDem_stCurr/1 -> Relational Operator/1
  VMD_trqDes/1 -> Switch/3, Add/1
  CrCtl_stSubGvnr/1 -> Relational Operator1/1
  Relational Operator1/1 -> Switch1/2
  CrCtl_stVDirChng/1 -> Switch/2
  Switch/1 -> Switch1/1
  Constant1/1 -> Relational Operator1/2
  Relational Operator/1 -> Switch2/2
  Add/1 -> Switch/1
  PT_trqWhlMinEng/1 -> Switch1/3
  Switch1/1 -> Switch2/3
  PT_rTraV2N/1 -> CrCtl_rTraV2NBeg/1
  Saturation_S16/1 -> CrCtl_trqReq/1, Switch3/3, Add3/1
  CrCtl_stGearRng_mp/1 -> Parameter Selection for Kp/1(CrCtl_stGearRng_mp)
  Parameter Selection for Kp/2(Out2) -> P_S16/3
  Add3/1 -> Switch3/1
  GlbDa_vXFlt/1 -> Add1/2, Add2/2
  CrCtl_facTipUpCor_CUR/1 -> Product/2
  GlbDa_aXFlt/1 -> CrCtl_facTipUpCor_CUR/1
  Parameter Selection for Kp/5(Out5) -> P_S16/6
  Constant2/1 -> Switch3/2
  Switch3/1 -> CrCtl_trqReqIWin_mp/1
  Switch2/1 -> Saturation_S16/1
  CrCtl_trqTipUpVDvtnCor_CUR/1 -> Product/1
  Product/1 -> Add/2  "CrCtl_trqTipUpCor_mp"
  Add2/1 -> P_S16/1
  Parameter Selection for Kp/1(Out1) -> P_S16/2
  Parameter Selection for Kp/3(Out3) -> P_S16/4
  CrCtl_vDesAct/1 -> Add2/1
  CrCtl_trqLimAct/1 -> Saturation_S16/3
  PT_trqWhl/1 -> Switch2/1
  CrCtl_trqMin/1 -> Saturation_S16/2
  CrCtl_vDesActOld/1 -> Add1/1
  Parameter Selection for Kp/4(Out4) -> P_S16/5
  Add1/1 -> CrCtl_trqTipUpVDvtnCor_CUR/1  "CrCtl_vDiffOldRfncSpd_mp"
  P_S16/1 -> CrCtl_trqReqPWin_mp/1, Add3/2

== system CrCtl_Governor/Working Range of Cruise Control/Lower limiting Cruise Control torque ==
  PT_trqWhlMinEngBrk : Inport
  PT_trqWhlMinEng : Inport  Port=2
  stvHysEngBrkReq : Inport  Port=3
  EBrk_stPreSelMode : Inport  Port=4
  Add : Sum
  Constant : Constant  Value=CrCtl_swtBrkMode_C
  Constant1 : Constant  OutDataTypeStr=State_uint8
  Constant2 : Constant  Value=EBrk_stPreSelMode_conv.EBPRESEL_STEB_SRVBRKFULL
  Constant3 : Constant  Value=EBrk_stPreSelMode_conv.EBPRESEL_STEB_SRVBRK50
  Constant4 : Constant  Value=TRQPRPHIGH_ZERO  OutDataTypeStr=Trq_Nm
  Logical Operator : Logic  Operator=OR  AllPortsSameDT=off  OutDataTypeStr=boolean
  Multiport Switch : MultiPortSwitch  Inputs=5
  Relational Operator : RelationalOperator  Operator===  OutDataTypeStr=boolean  RndMeth=Simplest
  Relational Operator1 : RelationalOperator  Operator===  OutDataTypeStr=boolean  RndMeth=Simplest
  Switch : Switch  Criteria=u2 ~= 0
  Switch1 : Switch  Criteria=u2 ~= 0
  CrCtl_trqMin : Outport
  wires:
  EBrk_stPreSelMode/1 -> Relational Operator1/1, Relational Operator/1
  Logical Operator/1 -> Switch1/2
  Constant2/1 -> Relational Operator/2
  Constant1/1 -> Add/2
  Constant/1 -> Add/1
  Relational Operator1/1 -> Logical Operator/2
  Constant3/1 -> Relational Operator1/2
  Multiport Switch/1 -> CrCtl_trqMin/1
  Constant4/1 -> Multiport Switch/6
  PT_trqWhlMinEngBrk/1 -> Switch1/1, Multiport Switch/3, Switch/1
  Switch1/1 -> Multiport Switch/4
  Relational Operator/1 -> Logical Operator/1
  Switch/1 -> Multiport Switch/5
  PT_trqWhlMinEng/1 -> Switch1/3, Multiport Switch/2, Switch/3
  Add/1 -> Multiport Switch/1
  stvHysEngBrkReq/1 -> Switch/2

== system CrCtl_Governor/Working Range of Cruise Control/Upper limiting Cruise Control torque ==
  CrCtl_trqMin : Inport
  stvHysEngBrkReq : Inport  Port=2
  PT_trqWhlMinEng : Inport  Port=3
  InjSys_trqLim : Inport  Port=4
  EngDem_trqInrLim : Inport  Port=5
  CoETS_trqUnFltLtd : Inport  Port=6
  CoETS_trqNTCActvOff : Inport  Port=7
  CoETS_trqNTCActvOn : Inport  Port=8
  RngMod_trqMin : Inport  Port=9
  PT_trqLos : Inport  Port=10
  PT_rTrq : Inport  Port=11
  VehMot_rTrqDfftl : Inport  Port=12
  CoVeh_trqAcs : Inport  Port=13
  CoVeh_trqPrpLimErr : Inport  Port=14
  Add{,2..4} (4 alike) : Sum  Inputs=+-
  Add1 : Sum
  Constant : Constant  Value=CrCtl_trqEngBrkOffOfs_C
  Constant1 : Constant  Value=0.0  OutDataTypeStr=Trq_Nm
  MinMax : MinMax  Inputs=2
  MinMax1 : MinMax  Inputs=2
  MinMax2 : MinMax  Inputs=2
  Product : Product  OutDataTypeStr=Trq_Nm  RndMeth=Nearest
  Product2 : Product  OutDataTypeStr=Trq_Nm
  Relational Operator : RelationalOperator  Operator=<  OutDataTypeStr=boolean  RndMeth=Simplest
  Switch : Switch  Criteria=u2 ~= 0
  Switch1 : Switch  Criteria=u2 ~= 0
  CrCtl_trqLimAct : Outport
  wires:
  InjSys_trqLim/1 -> MinMax/1
  EngDem_trqInrLim/1 -> MinMax/2
  MinMax/1 -> Add/1
  CoETS_trqUnFltLtd/1 -> Add/2
  stvHysEngBrkReq/1 -> Switch/2
  Add/1 -> Switch/3
  PT_trqWhlMinEng/1 -> Relational Operator/2
  CrCtl_trqMin/1 -> Relational Operator/1
  Relational Operator/1 -> Switch1/2
  CoETS_trqNTCActvOn/1 -> Switch1/3
  CoETS_trqNTCActvOff/1 -> Add1/1
  Constant/1 -> Add1/2
  Add1/1 -> MinMax1/1
  Constant1/1 -> MinMax1/2
  MinMax1/1 -> Switch1/1
  Switch1/1 -> Switch/1
  RngMod_trqMin/1 -> Add2/2
  Add2/1 -> Add3/1
  PT_trqLos/1 -> Add3/2
  Add3/1 -> Add4/1
  CoVeh_trqAcs/1 -> Add4/2
  Add4/1 -> Product/1
  PT_rTrq/1 -> Product/2
  Product/1 -> MinMax2/1
  CoVeh_trqPrpLimErr/1 -> MinMax2/2
  MinMax2/1 -> Product2/1
  VehMot_rTrqDfftl/1 -> Product2/2
  Product2/1 -> CrCtl_trqLimAct/1
  Switch/1 -> Add2/1

== system CrCtl_Governor/Acceleration State/CRCTL_SUBRMP/CrCtl_OverRide ==
  CrCtl_trqLimAct : Inport
  CrCtl_trqMin : Inport  Port=2
  APP_r : Inport  Port=3
  AccPed_trqDes : Inport  Port=4
  CrCtl_vDes : Inport  Port=5
  GlbDa_vXFlt : Inport  Port=6
  CrCtl_trqReq : Inport  Port=7
  CrCtl_trqIWinOld_mp : Inport  Port=8
  Add : Sum
  Bit Clear : simulink/Logic and Bit Operations/Bit Clear  iBit=1
  Bit Clear7 : simulink/Logic and Bit Operations/Bit Clear  iBit=0
  Bit Set : simulink/Logic and Bit Operations/Bit Set  iBit=1
  Bit Set7 : simulink/Logic and Bit Operations/Bit Set  iBit=0
  Constant : Constant  Value=0
  Constant2 : Constant  Value=CrCtl_vCnclOverride_C
  Constant8 : Constant  Value=CrCtl_swtOvrRdeFrzInteg_C
  Logical Operator : Logic  AllPortsSameDT=off  OutDataTypeStr=boolean
  Logical Operator1 : Logic  AllPortsSameDT=off  OutDataTypeStr=boolean
  Relational Operator : RelationalOperator  Operator=>  OutDataTypeStr=boolean  RndMeth=Simplest
  Relational Operator1 : RelationalOperator  Operator=>  OutDataTypeStr=boolean  RndMeth=Simplest
  Relational Operator2 : RelationalOperator  Operator=<=  OutDataTypeStr=boolean  RndMeth=Simplest
  Relational Operator3 : RelationalOperator  Operator=<  OutDataTypeStr=boolean  RndMeth=Simplest
  Saturation_S16 : CXLib/Saturation_S16
  Switch : Switch  Criteria=u2 ~= 0
  Switch7 : Switch  Criteria=u2 ~= 0
  Switch8 : Switch  Criteria=u2 ~= 0
  Terminator1 : Terminator
  Unit Delay : UnitDelay  SampleTime=-1
  CrCtl_stIWin_mp : Outport
  CrCtl_trqReqIWin_mp : Outport  Port=2
  wires:
  APP_r/1 -> Relational Operator/1
  Constant/1 -> Relational Operator/2
  AccPed_trqDes/1 -> Relational Operator1/1, Relational Operator2/1
  Relational Operator/1 -> Logical Operator/1
  Relational Operator1/1 -> Logical Operator/2
  Logical Operator/1 -> Switch/2
  Relational Operator2/1 -> Logical Operator1/1
  Relational Operator3/1 -> Logical Operator1/2
  GlbDa_vXFlt/1 -> Relational Operator3/1
  CrCtl_vDes/1 -> Add/1
  Add/1 -> Relational Operator3/2
  Constant2/1 -> Add/2
  CrCtl_trqLimAct/1 -> Saturation_S16/3
  CrCtl_trqMin/1 -> Saturation_S16/2
  Bit Set/1 -> Switch/1
  Bit Clear/1 -> Switch/3
  Switch/1 -> Bit Clear7/1, Bit Set7/1
  Constant8/1 -> Switch7/2
  Bit Set7/1 -> Switch7/1
  Bit Clear7/1 -> Switch7/3
  Switch7/1 -> CrCtl_stIWin_mp/1, Unit Delay/1
  Unit Delay/1 -> Bit Set/1, Bit Clear/1
  CrCtl_trqReq/1 -> Saturation_S16/1
  Saturation_S16/1 -> Switch8/3, Relational Operator2/2, Relational Operator1/2
  Saturation_S16/2 -> Terminator1/1
  Logical Operator1/1 -> Switch8/2
  CrCtl_trqIWinOld_mp/1 -> Switch8/1
  Switch8/1 -> CrCtl_trqReqIWin_mp/1

== system CrCtl_Governor/Acceleration State/CRCTL_SUBRMP/CrCtl_Suspend ==
  PT_trqWhlMinEng : Inport
  CrCtl_trqReqOld : Inport  Port=2
  AccPed_trqDes : Inport  Port=3
  CrCtl_trqLimAct : Inport  Port=4
  CrCtl_stSuspAct : Inport  Port=5
  Constant : Constant  Value=true
  Constant1 : Constant  Value=CrCtl_stSuspRamp_conv.CRCTL_SUSPENDENDRAMP
  Constant2 : Constant  Value=CrCtl_stSuspRamp_conv.CRCTL_SUSPENDRAMPDONE
  Constant3 : Constant  Value=CrCtl_stSuspRamp_conv.CRCTL_SUSPENDNOTACTIVE
  Constant4 : Constant  Value=CrCtl_stSuspRamp_conv.CRCTL_SUSPENDSTARTRAMP
  EdgeFalling : CXLib/EdgeFalling
  EdgeRising : CXLib/EdgeRising
  EdgeRising1 : CXLib/EdgeRising
  Logical Operator : Logic  Operator=NOT  AllPortsSameDT=off  OutDataTypeStr=boolean
  Subsystem : Subsystem
  Subsystem1 : Subsystem
  Switch{,1..3,5} (5 alike) : Switch  Criteria=u2 ~= 0
  Unit Delay : UnitDelay  SampleTime=-1
  CrCtl_stSuspRamp : Outport
  " CrCtl_trqReq" : Outport  Port=2
  wires:
  Subsystem/1(Out) -> Switch1/2, Subsystem1/5(In1)
  Subsystem/2(Out1) -> Switch5/1, Subsystem1/6(In2)
  PT_trqWhlMinEng/1 -> Subsystem/1(PT_trqWhlMinEng), Subsystem1/1(PT_trqWhlMinEng)
  CrCtl_trqReqOld/1 -> Subsystem/2(CrCtl_trqReqOld), Subsystem1/2(CrCtl_trqReqOld)
  CrCtl_trqLimAct/1 -> Subsystem1/4(CrCtl_trqLimAct)
  AccPed_trqDes/1 -> Subsystem1/3(AccPed_trqDes)
  Switch1/1 -> Switch/1
  Switch2/1 -> Switch/3
  Constant4/1 -> Switch1/1
  Constant2/1 -> Switch1/3
  Constant1/1 -> Switch2/1
  Constant3/1 -> Switch2/3
  Switch/1 -> CrCtl_stSuspRamp/1
  Subsystem1/1(Out1) -> Switch2/2
  Switch5/1 -> " CrCtl_trqReq"/1
  Subsystem1/2(Out2) -> Switch5/3
  Logical Operator/1 -> EdgeRising1/1
  EdgeRising/1 -> Subsystem/3(CrCtl_stSuspAct)
  EdgeRising1/1 -> Subsystem1/7(In3)
  CrCtl_stSuspAct/1 -> EdgeFalling/1, Logical Operator/1, Subsystem/Enable, Switch/2, Switch5/2, EdgeRising/1
  Constant/1 -> Switch3/1
  EdgeFalling/1 -> Switch3/2
  Switch3/1 -> Unit Delay/1, Subsystem1/Enable
  Unit Delay/1 -> Switch3/3

== system CrCtl_Governor/Acceleration State/CRCTL_SUBRMP/Governor ==
  CrCtl_trqLimAct : Inport
  CrCtl_trqMin : Inport  Port=2
  CrCtl_stGearRng_mp : Inport  Port=3
  CrCtl_vDesAct : Inport  Port=4
  stvHysEngBrkReq : Inport  Port=5
  GlbDa_vXFlt : Inport  Port=6
  stCrCtlOn : Inport  Port=7
  In1 : Inport  Port=8
  In2 : Inport  Port=9
  Enable : EnablePort
  Add1 : Sum  Inputs=+-
  Add2 : Sum
  Add3 : Sum  OutDataTypeStr=Trq_Nm
  Constant : Constant  Value=CrCtl_swtILimWithP_C
  Constant1 : Constant  Value=CrCtl_Governor_DT
  Constant2 : Constant  Value=1000  OutDataTypeStr=Inherit: Inherit via back propagation
  CrCtl_ARW : Subsystem
  I_S16 : CXLib/I_S16
  PT1 Filtered Torque : Subsystem
  P_S16 : CXLib/P_S16
  Parameter Selection for Ki : Subsystem
  Parameter Selection for Kp : Subsystem
  Product : Product  OutDataTypeStr=uint32
  Saturation_S16 : CXLib/Saturation_S16
  Switch : Switch  Criteria=u2 ~= 0
  Terminator : Terminator
  Unit Delay : UnitDelay  SampleTime=-1
  Unit Delay1 : UnitDelay  SampleTime=-1
  CrCtl_trqReq : Outport
  CrCtl_trqIWinOld_mp : Outport  Port=2  OutDataTypeStr=Trq_Nm
  CrCtl_trqReqPWin_mp : Outport  Port=3
  wires:
  CrCtl_vDesAct/1 -> Add1/1
  GlbDa_vXFlt/1 -> Add1/2
  Add1/1 -> P_S16/1, I_S16/1, PT1 Filtered Torque/2(vDiffCrCtl)
  Add2/1 -> Add3/1
  Add3/1 -> Saturation_S16/1
  CrCtl_trqMin/1 -> CrCtl_ARW/2(CrCtl_trqMin), Saturation_S16/2
  CrCtl_trqLimAct/1 -> CrCtl_ARW/3(CrCtl_trqLimAct), Saturation_S16/3
  Saturation_S16/2 -> Terminator/1
  Saturation_S16/1 -> CrCtl_trqReq/1
  Switch/1 -> CrCtl_ARW/5(CrCtl_trqReqIWin_mp), CrCtl_trqIWinOld_mp/1, Add2/2
  P_S16/1 -> CrCtl_trqReqPWin_mp/1, CrCtl_ARW/4(CrCtl_trqReqPWin_mp), Add2/1
  Constant/1 -> CrCtl_ARW/1(CrCtl_swtILimWithP_C)
  stvHysEngBrkReq/1 -> PT1 Filtered Torque/1(stvHysEngBrkReq)
  CrCtl_stGearRng_mp/1 -> PT1 Filtered Torque/3(CrCtl_stGearRng_mp), Parameter Selection for Ki/1(CrCtl_stGearRng_mp), Parameter Selection for Kp/1(CrCtl_stGearRng_mp)
  stCrCtlOn/1 -> PT1 Filtered Torque/4(stCrCtlOn)
  Parameter Selection for Kp/1(Out1) -> P_S16/2
  Parameter Selection for Kp/2(Out2) -> P_S16/3
  Parameter Selection for Kp/3(Out3) -> P_S16/4
  Parameter Selection for Kp/4(Out4) -> P_S16/5
  Parameter Selection for Kp/5(Out5) -> P_S16/6
  Parameter Selection for Ki/1(Out1) -> I_S16/3
  Parameter Selection for Ki/2(Out2) -> I_S16/4
  Parameter Selection for Ki/3(Out3) -> I_S16/5
  Parameter Selection for Ki/5(Out5) -> I_S16/7
  CrCtl_ARW/2(Limit) -> Unit Delay1/1
  CrCtl_ARW/1(CrCtl_stInit_mp) -> Unit Delay/1  "CrCtl_stInit_mp"
  Product/1 -> I_S16/2
  Constant2/1 -> Product/2
  Constant1/1 -> Product/1
  PT1 Filtered Torque/1(CrCtl_trqDesvHys) -> Add3/2
  I_S16/1 -> Switch/3
  Unit Delay1/1 -> Switch/1
  Unit Delay/1 -> Switch/2
  In1/1 -> I_S16/8
  In2/1 -> I_S16/9
  Parameter Selection for Ki/4(Out4) -> I_S16/6

== system CrCtl_Governor/Cruise State/CRCTL_SUBGVNR/CrCtl_OverRide ==
  CrCtl_trqLimAct : Inport
  CrCtl_trqMin : Inport  Port=2
  APP_r : Inport  Port=3
  AccPed_trqDes : Inport  Port=4
  CrCtl_vDes : Inport  Port=5
  GlbDa_vXFlt : Inport  Port=6
  CrCtl_trqReq : Inport  Port=7
  CrCtl_trqIWinOld_mp : Inport  Port=8
  Add : Sum
  Bit Clear : simulink/Logic and Bit Operations/Bit Clear  iBit=1
  Bit Clear7 : simulink/Logic and Bit Operations/Bit Clear  iBit=0
  Bit Set : simulink/Logic and Bit Operations/Bit Set  iBit=1
  Bit Set7 : simulink/Logic and Bit Operations/Bit Set  iBit=0
  Constant : Constant  Value=0
  Constant2 : Constant  Value=CrCtl_vCnclOverride_C
  Constant8 : Constant  Value=CrCtl_swtOvrRdeFrzInteg_C
  Logical Operator : Logic  AllPortsSameDT=off  OutDataTypeStr=boolean
  Logical Operator1 : Logic  AllPortsSameDT=off  OutDataTypeStr=boolean
  Relational Operator : RelationalOperator  Operator=>  OutDataTypeStr=boolean  RndMeth=Simplest
  Relational Operator1 : RelationalOperator  Operator=>  OutDataTypeStr=boolean  RndMeth=Simplest
  Relational Operator2 : RelationalOperator  Operator=<=  OutDataTypeStr=boolean  RndMeth=Simplest
  Relational Operator3 : RelationalOperator  Operator=<  OutDataTypeStr=boolean  RndMeth=Simplest
  Saturation_S16 : CXLib/Saturation_S16
  Switch : Switch  Criteria=u2 ~= 0
  Switch7 : Switch  Criteria=u2 ~= 0
  Switch8 : Switch  Criteria=u2 ~= 0
  Terminator1 : Terminator
  Unit Delay : UnitDelay  SampleTime=-1
  CrCtl_stIWin_mp : Outport
  CrCtl_trqReqIWin_mp : Outport  Port=2
  wires:
  APP_r/1 -> Relational Operator/1
  Constant/1 -> Relational Operator/2
  AccPed_trqDes/1 -> Relational Operator1/1, Relational Operator2/1
  Relational Operator/1 -> Logical Operator/1
  Relational Operator1/1 -> Logical Operator/2
  Logical Operator/1 -> Switch/2
  Relational Operator2/1 -> Logical Operator1/1
  Relational Operator3/1 -> Logical Operator1/2
  GlbDa_vXFlt/1 -> Relational Operator3/1
  CrCtl_vDes/1 -> Add/1
  Add/1 -> Relational Operator3/2
  Constant2/1 -> Add/2
  CrCtl_trqLimAct/1 -> Saturation_S16/3
  CrCtl_trqMin/1 -> Saturation_S16/2
  Bit Set/1 -> Switch/1
  Bit Clear/1 -> Switch/3
  Switch/1 -> Bit Clear7/1, Bit Set7/1
  Constant8/1 -> Switch7/2
  Bit Set7/1 -> Switch7/1
  Bit Clear7/1 -> Switch7/3
  Switch7/1 -> CrCtl_stIWin_mp/1, Unit Delay/1
  Unit Delay/1 -> Bit Set/1, Bit Clear/1
  CrCtl_trqReq/1 -> Saturation_S16/1
  Saturation_S16/1 -> Switch8/3, Relational Operator2/2, Relational Operator1/2
  Saturation_S16/2 -> Terminator1/1
  Logical Operator1/1 -> Switch8/2
  CrCtl_trqIWinOld_mp/1 -> Switch8/1
  Switch8/1 -> CrCtl_trqReqIWin_mp/1
